simulink subsystem "rss_BusOffFaltDia"  (R2023a)
settings: Solver=VariableStepAuto  StartTime=0.0  StopTime=10.0  RelTol=1e-3
undefined symbols (not defined in the file): ENM_TYPE_FALT, Gu16_ctBusOffFaltConfCnt_C, Gu16_ctBusOffFaltRcvyCnt_C
libraries: lib_debounce x1, lib_fault_definiteness x1
settings Model: Creator=xiaoqiang.yuan  LastModifiedBy=xiaoqiang.yuan

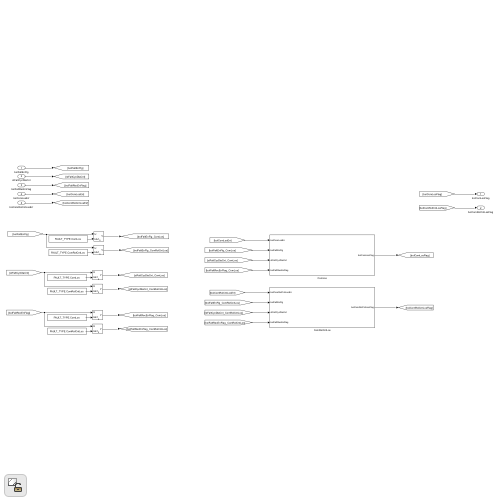
[thumbnail: Simulink's stored preview of the top-level diagram]
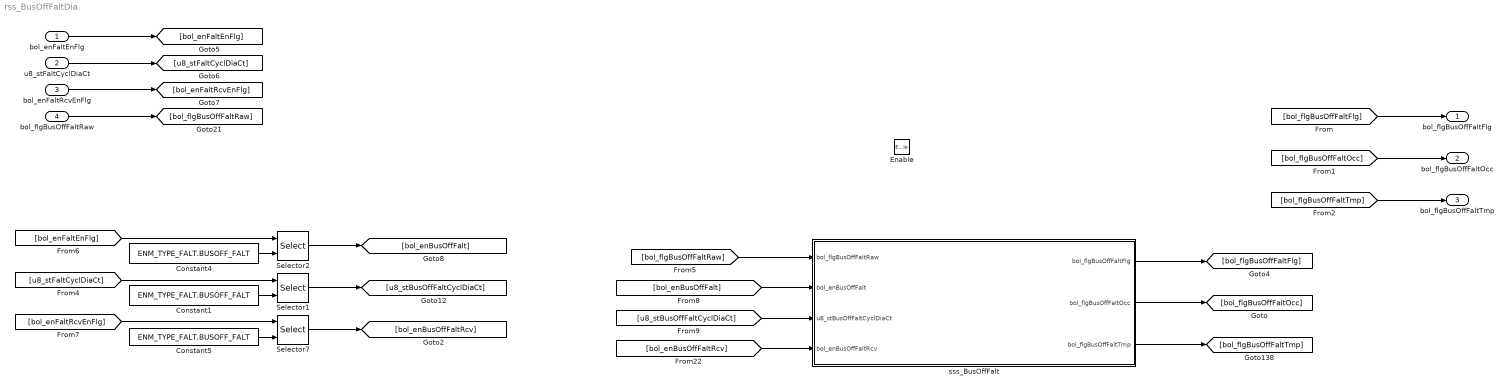
== system rss_BusOffFaltDia ==
  bol_enFaltEnFlg : Inport  OutDataTypeStr=boolean
  u8_stFaltCyclDiaCt : Inport  Port=2  OutDataTypeStr=uint8
  bol_enFaltRcvEnFlg : Inport  Port=3  OutDataTypeStr=boolean
  bol_flgBusOffFaltRaw : Inport  Port=4  OutDataTypeStr=boolean
  Enable : EnablePort
  Constant1 : Constant  Value=ENM_TYPE_FALT.BUSOFF_FALT
  Constant4 : Constant  Value=ENM_TYPE_FALT.BUSOFF_FALT
  Constant5 : Constant  Value=ENM_TYPE_FALT.BUSOFF_FALT
  Selector1 : Selector  IndexMode=Zero-based  InputPortWidth=Cdbl_numFaltDiaNum  IndexOptions=Index vector (port)  Indices=[1 3]  OutputSizes=1
  Selector2 : Selector  IndexMode=Zero-based  InputPortWidth=Cdbl_numFaltDiaNum  IndexOptions=Index vector (port)  Indices=[1 3]  OutputSizes=1
  Selector7 : Selector  IndexMode=Zero-based  InputPortWidth=Cdbl_numFaltDiaNum  IndexOptions=Index vector (port)  Indices=[1 3]  OutputSizes=1
  sss_BusOffFalt : Subsystem
  bol_flgBusOffFaltFlg : Outport  OutDataTypeStr=boolean
  bol_flgBusOffFaltOcc : Outport  Port=2  OutDataTypeStr=boolean
  bol_flgBusOffFaltTmp : Outport  Port=3  OutDataTypeStr=boolean
  wires:
  [bol_flgBusOffFaltFlg] -> bol_flgBusOffFaltFlg/1
  [bol_flgBusOffFaltOcc] -> bol_flgBusOffFaltOcc/1
  [u8_stFaltCyclDiaCt] -> Selector1/1
  [bol_enFaltEnFlg] -> Selector2/1
  bol_enFaltEnFlg/1 -> [bol_enFaltEnFlg]
  bol_enFaltRcvEnFlg/1 -> [bol_enFaltRcvEnFlg]
  [bol_flgBusOffFaltRaw] -> sss_BusOffFalt/1(bol_flgBusOffFaltRaw)
  Constant1/1 -> Selector1/2
  [u8_stBusOffFaltCyclDiaCt] -> sss_BusOffFalt/3(u8_stBusOffFaltCyclDiaCt)
  [bol_enBusOffFalt] -> sss_BusOffFalt/2(bol_enBusOffFalt)
  Constant4/1 -> Selector2/2
  Constant5/1 -> Selector7/2
  Selector1/1 -> [u8_stBusOffFaltCyclDiaCt]
  bol_flgBusOffFaltRaw/1 -> [bol_flgBusOffFaltRaw]
  Selector7/1 -> [bol_enBusOffFaltRcv]
  [bol_enFaltRcvEnFlg] -> Selector7/1
  Selector2/1 -> [bol_enBusOffFalt]
  [bol_enBusOffFaltRcv] -> sss_BusOffFalt/4(bol_enBusOffFaltRcv)
  u8_stFaltCyclDiaCt/1 -> [u8_stFaltCyclDiaCt]
  sss_BusOffFalt/1(bol_flgBusOffFaltFlg) -> [bol_flgBusOffFaltFlg]
  sss_BusOffFalt/2(bol_flgBusOffFaltOcc) -> [bol_flgBusOffFaltOcc]
  [bol_flgBusOffFaltTmp] -> bol_flgBusOffFaltTmp/1
  sss_BusOffFalt/3(bol_flgBusOffFaltTmp) -> [bol_flgBusOffFaltTmp]

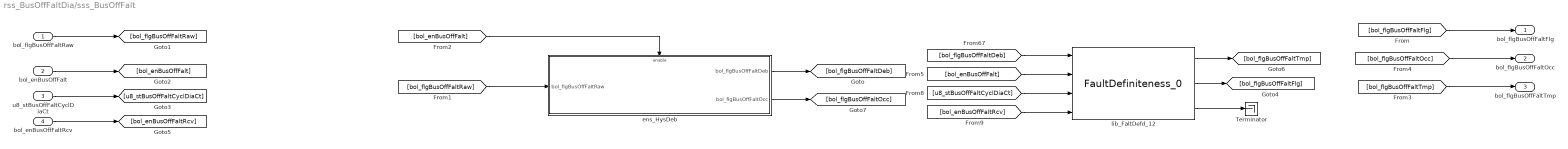
== system rss_BusOffFaltDia/sss_BusOffFalt ==
  bol_flgBusOffFaltRaw : Inport
  bol_enBusOffFalt : Inport  Port=2
  u8_stBusOffFaltCyclDiaCt : Inport  Port=3
  bol_enBusOffFaltRcv : Inport  Port=4
  Terminator : Terminator
  ens_HysDeb : Subsystem
  lib_FaltDefd_12 : lib_fault_definiteness/FaultDefiniteness_0  lb_FaltWaitRecvCnt=Gu16_ctBusOffFaltConfCnt_C
  bol_flgBusOffFaltFlg : Outport
  bol_flgBusOffFaltOcc : Outport  Port=2
  bol_flgBusOffFaltTmp : Outport  Port=3
  wires:
  [bol_flgBusOffFaltTmp] -> bol_flgBusOffFaltTmp/1
  [bol_flgBusOffFaltRaw] -> ens_HysDeb/1(bol_flgBusOffFaltRaw)
  [bol_flgBusOffFaltOcc] -> bol_flgBusOffFaltOcc/1
  ens_HysDeb/2(bol_flgBusOffFaltOcc) -> [bol_flgBusOffFaltOcc]
  lib_FaltDefd_12/1 -> [bol_flgBusOffFaltTmp]
  lib_FaltDefd_12/2 -> [bol_flgBusOffFaltFlg]
  lib_FaltDefd_12/3 -> Terminator/1
  [bol_enBusOffFalt] -> ens_HysDeb/Enable
  ens_HysDeb/1(bol_flgBusOffFaltDeb) -> [bol_flgBusOffFaltDeb]
  bol_enBusOffFaltRcv/1 -> [bol_enBusOffFaltRcv]
  u8_stBusOffFaltCyclDiaCt/1 -> [u8_stBusOffFaltCyclDiaCt]
  bol_enBusOffFalt/1 -> [bol_enBusOffFalt]
  [bol_flgBusOffFaltFlg] -> bol_flgBusOffFaltFlg/1
  bol_flgBusOffFaltRaw/1 -> [bol_flgBusOffFaltRaw]
  [bol_enBusOffFaltRcv] -> lib_FaltDefd_12/4
  [u8_stBusOffFaltCyclDiaCt] -> lib_FaltDefd_12/3
  [bol_enBusOffFalt] -> lib_FaltDefd_12/2
  [bol_flgBusOffFaltDeb] -> lib_FaltDefd_12/1

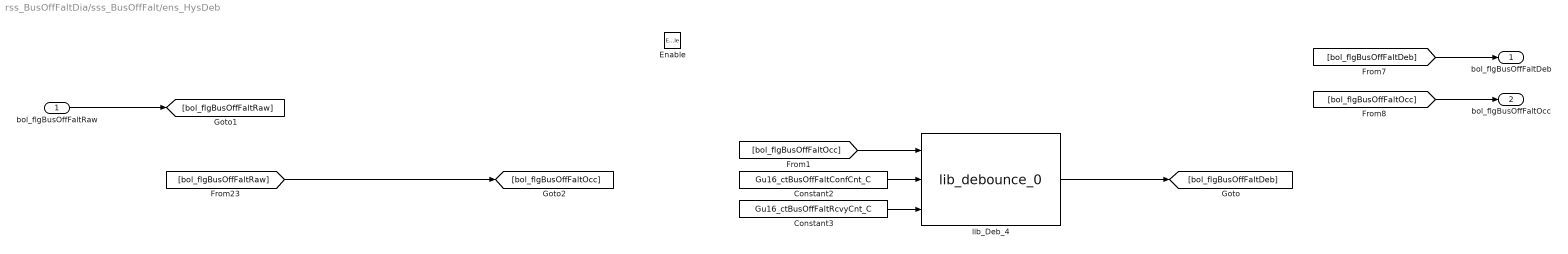
== system rss_BusOffFaltDia/sss_BusOffFalt/ens_HysDeb ==
  bol_flgBusOffFaltRaw : Inport
  Enable : EnablePort
  Constant2 : Constant  Value=Gu16_ctBusOffFaltConfCnt_C
  Constant3 : Constant  Value=Gu16_ctBusOffFaltRcvyCnt_C
  lib_Deb_4 : lib_debounce/lib_debounce_0
  bol_flgBusOffFaltDeb : Outport
  bol_flgBusOffFaltOcc : Outport  Port=2
  wires:
  [bol_flgBusOffFaltOcc] -> bol_flgBusOffFaltOcc/1
  [bol_flgBusOffFaltOcc] -> lib_Deb_4/1
  [bol_flgBusOffFaltRaw] -> [bol_flgBusOffFaltOcc]
  lib_Deb_4/1 -> [bol_flgBusOffFaltDeb]
  bol_flgBusOffFaltRaw/1 -> [bol_flgBusOffFaltRaw]
  [bol_flgBusOffFaltDeb] -> bol_flgBusOffFaltDeb/1
  Constant3/1 -> lib_Deb_4/3
  Constant2/1 -> lib_Deb_4/2
